simulink model "velfb"  (R2015a)
settings: Solver=ode45  StartTime=0.0  StopTime=10.0  RelTol=1e-3
values from neighbouring files (symbols this model uses):
  Kt = 0.5    [velfb.m]
undefined symbols (not defined in the file or in its folder): K
settings Model: ExtModeTrigMode=oneshot  ExtModeArmWhenConnect=off  Creator=eechris  LastModifiedBy=eechris
settings DataIOCC: LimitDataPoints=off  SignalLoggingSaveFormat=ModelDataLogs
settings OptimizationCC: BlockReduction=off  BooleanDataType=off
settings DebuggingCC: SaveWithParameterizedLinksMsg=none  UnderspecifiedInitializationDetection=Classic  MergeDetectMultiDrivingBlocksExec=none  SignalResolutionControl=TryResolveAllWithWarning  MultiTaskDSMMsg=warning  MultiTaskCondExecSysMsg=none  StrictBusMsg=None
settings HardwareCC: TargetUnknown=on
settings GRTTargetCC: CombineOutputUpdateFcns=off  GRTInterface=on

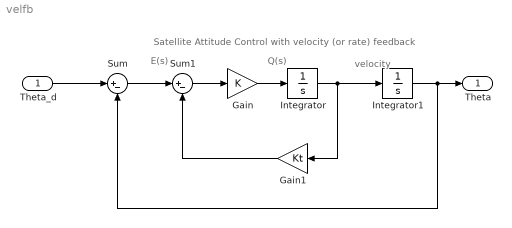
== system velfb ==
  note: Satellite Attitude Control with velocity (or rate) feedback
  note: E(s)
  note: Q(s)
  note: velocity
  Theta_d : Inport
  Gain : Gain  Gain=K  SaturateOnIntegerOverflow=on  OutDataTypeStr=Inherit: Same as input  ParamDataTypeStr=Inherit: Same as input
  Gain1 : Gain  Gain=Kt  SaturateOnIntegerOverflow=on  OutDataTypeStr=Inherit: Same as input  ParamDataTypeStr=Inherit: Same as input
  Integrator : Integrator
  Integrator1 : Integrator
  Sum : Sum  Inputs=|+-  SaturateOnIntegerOverflow=on  InputSameDT=on  OutDataTypeStr=Inherit: Same as first input
  Sum1 : Sum  Inputs=|+-  SaturateOnIntegerOverflow=on  InputSameDT=on  OutDataTypeStr=Inherit: Same as first input
  Theta : Outport
  wires:
  Gain/1 -> Integrator/1
  Sum1/1 -> Gain/1
  Theta_d/1 -> Sum/1
  Sum/1 -> Sum1/1
  Integrator/1 -> Integrator1/1, Gain1/1
  Gain1/1 -> Sum1/2
  Integrator1/1 -> Theta/1, Sum/2
